simulink model "wind_turbine_modified"  (R2023a)
settings: Solver=VariableStepAuto  StartTime=0.0  StopTime=10.0  RelTol=1e-3
undefined symbols (not defined in the file): F, find_system, Fnom, gcbh, H, ILd_init, ILq_init, Imax_grid_conv, Init, j, Ki_dc_reg, Ki_grid_side_cur_reg, Ki_power_reg, Ki_Q, Ki_rotor_side_cur_reg, Ki_volt_reg, Kp_dc_reg, Kp_grid_side_cur_reg, Kp_power_reg, Kp_Q, Kp_rotor_side_cur_reg, Kp_volt_reg, L_RL, Llr, Lls, p, Pnom, power_A, power_B, power_D, R_RL, Rr, Rs, speed_A, speed_B, speed_C, speed_D, sps_rtmsupport, Vcontrol, Vnom, Wind_On
libraries: simulink_extras x5, spsControlledCurrentSourceLib x4, spsThreePhaseVIMeasurementLib x2, spsWindTurbineDoublyFedInductionGeneratorPhasorTypeLib x1, spsBistableLib x1, spsPower3phPhasorLib x1, spsWindTurbineLib x1
(part 1 of 3)
settings Model: Creator=Adham  LastModifiedBy=Adham

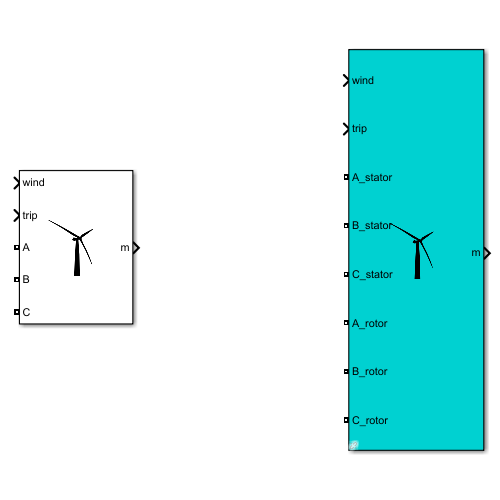
[thumbnail: Simulink's stored preview of the top-level diagram]
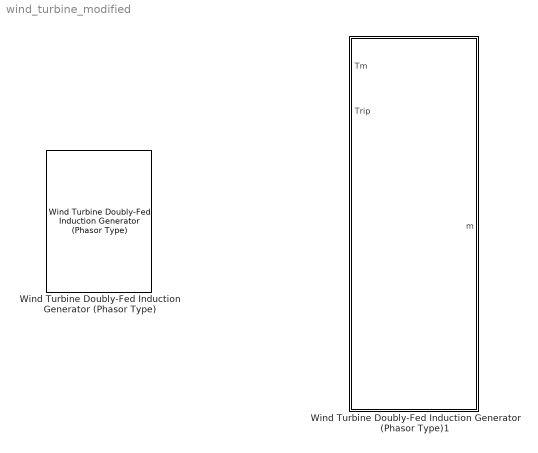
== system wind_turbine_modified ==
  Wind Turbine Doubly-Fed Induction Generator (Phasor Type) : spsWindTurbineDoublyFedInductionGeneratorPhasorTypeLib/Wind Turbine Doubly-Fed Induction Generator (Phasor Type)  ExternalTm=off  nom=[1.5e6/0.9 575 60]  sta=[ 0.00706 0.171]  rot=[ 0.005 0.156]  Lm=2.90  mec=[5.04 0.01 3]  init=[0.2 0 0 0 0 0]  speed_power=[0 0; 0.24 0.007; 0.36 0.024; 0.6 0.112; 0.96 0.46; 1.2 0.898; 1.5 0.898]  Pmec=1.5e6  speed_ABCD=[0.7 0.71 1.2 1.21]  power_C=0.73  wind_point_C=12  pitch_gain=500  pitch_max=45  pitch_rate=2  Pmax=0.5  Lchoke=[0.15 0.15/100]  init_inductor=[0 90]  Vdc_nom=1200  capacitor=10000e-6  ControlVQ=Voltage regulation  Vref=1.0  ExternalVref=off  Qref=0  ExternalQref=on  Iq_ref=0  ExternalIqref=off  Kpi_volt_reg=[1.25 300]  Xs=0.02  Kpi_Q=[0.05 5]  Kpi_power_reg=[1 100]  Kpi_dc_reg=[0.002 0.05]  Kpi_grid_side_cur_reg=[1 100]  Kpi_rotor_side_cur_reg=[0.3 8]  V_slew_rate=100  Q_slew_rate=100  power_slew_rate=1  current_slew_rate=200
      settings: LibrarySourceBlock=|
      | sps_lib/Electrical Machines/Wind Turbine
      | Doubly-Fed Induction Generator
      | (Phasor Type)
  Wind Turbine Doubly-Fed Induction Generator (Phasor Type)1 : Subsystem  AncestorBlock=|  DialogController=POWERSYS.PowerSysDialog  LoadFcn=sps_rtmsupport('LoadFcn',gcbh); %find_system(gcs,'FollowLinks', 'on', 'LookUnderMasks', 'all');  StartFcn=sps_rtmsupport('StartFcn',gcbh);  StopFcn=sps_rtmsupport('StopFcn',gcbh);  mask(Wind Turbine Doubly-Fed Induction Generator (Phasor Type)){ExternalTm=off, nom=[1.5e6/0.9 575 60], sta=[ 0.00706 0.171], rot=[ 0.005 0.156], Lm=2.90, mec=[5.04 0.01 3], init=[0.2 0 0 0 0 0], speed_power=[0 0; 0.24 0.007; 0.36 0.024; 0.6 0.112; 0.96 0.46; 1.2 0.898; 1.5 0.898], Pmec=1.5e6, speed_ABCD=[0.7 0.71 1.2 1.21], power_C=0.73, wind_point_C=12, pitch_gain=500, pitch_max=45, pitch_rate=2, Pmax=0.5, Lchoke=[0.15 0.15/100], init_inductor=[0 90], Vdc_nom=1200, capacitor=10000e-6, ControlVQ=Voltage regulation, Vref=1.0, ExternalVref=off, Qref=0, ExternalQref=on, Iq_ref=0, ExternalIqref=off, Kpi_volt_reg=[1.25 300], Xs=0.02, Kpi_Q=[0.05 5], Kpi_power_reg=[1 100], Kpi_dc_reg=[0.002 0.05], Kpi_grid_side_cur_reg=[1 100], Kpi_rotor_side_cur_reg=[0.3 8], V_slew_rate=100, Q_slew_rate=100, power_slew_rate=1, current_slew_rate=200}
      | sps_lib/Electrical Machines/Wind Turbine
      | Doubly-Fed Induction Generator
      | (Phasor Type)
      mask prompts: ExternalTm "External turbine (Tm mechanical torque input)"; nom "Nominal power, line-to-line voltage, frequency [Pn(VA), Vn(Vrms), fn(Hz)]:"; sta "Stator [Rs, Lls] (pu):"; rot "Rotor [Rr', Llr' ] (pu):"; Lm "Magnetizing inductance Lm (pu):"; mec "Inertia constant, friction factor, and pairs of poles [H(s), F(pu),  p ]:"; init "Initial conditions [s,  th(deg),  Is(pu), ph_Is(deg),  Ir(pu),  ph_Ir(deg)]:"; speed_power "Electric power-speed characteristic: [wr1(pu) p1(pu); wr2(pu) p2(pu); ... ]"; Pmec "Nominal wind turbine mechanical output power (W):"; speed_ABCD "Tracking characteristic speeds: [speed_A(pu) ... speed_D(pu)]"; power_C "Power at point C (pu/mechanical power):"; wind_point_C "Wind speed at point C (m/s):"; pitch_gain "Pitch angle controller gain [Kp]:"; pitch_max "Maximum pitch angle (deg):"; pitch_rate "Maximum rate of change of pitch angle (deg/s):"; Pmax "Converter maximum power (pu):"; Lchoke "Grid-side coupling inductor [L (pu) R (pu)]:"; init_inductor "Coupling inductor initial current: [ IL(pu) ph_IL(deg)]"; Vdc_nom "Nominal DC bus voltage (V):"; capacitor "DC bus capacitor (F):"; ControlVQ "Mode:"; Vref "Reference grid voltage Vref (pu):"; ExternalVref "External"; Qref "Generated reactive power Qref (pu):"; ExternalQref "External"; Iq_ref "Grid-side converter generated reactive current reference (Iq_ref) (pu):"; ExternalIqref "External"; Kpi_volt_reg "Grid voltage regulator gains: [Kp Ki]"; Xs "Droop Xs (pu):"; Kpi_Q "Reactive power regulator gains: [Kp Ki]"; Kpi_power_reg "Power regulator gains: [Kp Ki]"; Kpi_dc_reg "DC bus voltage regulator gains: [Kp Ki]"; Kpi_grid_side_cur_reg "Grid-side converter current regulator gains: [Kp Ki]"; Kpi_rotor_side_cur_reg "Rotor-side converter current regulator gains: [Kp Ki]"; V_slew_rate "Maximum rate of change of reference grid voltage (pu/s):"; Q_slew_rate "Maximum rate of change of reference reactive power (pu/s):"; power_slew_rate "Maximum rate of change of reference power (pu/s):"; current_slew_rate "Maximum rate of change of converter  reference currents (pu/s):"
      mask help: Implements a phasor model of a doubly-fed induction generator driven by a wind turbine.
      mask init:
      | [Pnom,Vnom,Fnom,Rs,Lls,Rr,Llr,H,p,F,Wind_On,FACTSroot,mag_IL_init,ph_IL_init,ILd_init,ILq_init,Imax_grid_conv,speed_A,speed_B,speed_C,speed_D,power_A,power_B,power_D,L_RL,R_RL,Kp_volt_reg,Ki_volt_reg,Kp_Q,Ki_Q,Kp_power_reg,Ki_power_reg,Kp_dc_reg,Ki_dc_reg,Kp_grid_side_cur_reg,Ki_grid_side_cur_reg,Kp_rotor_side_cur_reg,Ki_rotor_side_cur_reg,Vcontrol] ...
      |     = WindTurbineInit (nom,sta,rot,mec,ExternalTm,1,gcbh,Pmax,Lchoke,init_inductor,speed_ABCD,power_C,Kpi_volt_reg,Kpi_Q,Kpi_power_reg,Kpi_dc_reg,Kpi_grid_side_cur_reg,Kpi_rotor_side_cur_reg,ControlVQ);
      settings: CopyFcn=sps_rtmsupport('CopyFcn',gcbh);  DeleteFcn=sps_rtmsupport('DeleteFcn',gcbh);  UndoDeleteFcn=sps_rtmsupport('UndoDeleteFcn',gcbh);  ModelCloseFcn=sps_rtmsupport('ModelCloseFcn',gcbh);  PreSaveFcn=sps_rtmsupport('PreSaveFcn',gcbh);  PostSaveFcn=sps_rtmsupport('PostSaveFcn',gcbh);  NameChangeFcn=sps_rtmsupport('NameChangeFcn',gcbh);  PreCopyFcn=sps_rtmsupport('PreCopyFcn',gcbh);  OpenFcn=sps_rtmsupport('OpenFcn',gcbh, [1 21,23,25,27]);  CloseFcn=sps_rtmsupport('CloseFcn',gcbh);  PreDeleteFcn=sps_rtmsupport('PreDeleteFcn',gcbh);
      settings: LibrarySourceBlock=|
      | sps_lib/Electrical Machines/Wind Turbine
      | Doubly-Fed Induction Generator
      | (Phasor Type)
      mask Help: helpview(psbhelp)
      mask Callback ExternalTm: WindTurbineCback(gcbh);
      mask TypeOptions ControlVQ: Voltage regulation | Var regulation
      mask Callback ControlVQ: WindTurbineCback(gcbh);
      mask Callback ExternalVref: WindTurbineCback(gcbh);
      mask Callback ExternalQref: WindTurbineCback(gcbh);
      mask Callback ExternalIqref: WindTurbineCback(gcbh);
      mask DialogControl generatordata Prompt: Generator
      mask DialogControl turbinedata Prompt: Turbine
      mask DialogControl Display Prompt: Display wind turbine power characteristics
      mask DialogControl Display Callback: WindTurbineDisplay(gcbh);
      mask DialogControl convertersdata Prompt: Converters
      mask DialogControl controlparameters Prompt: Control
      mask Display:
      | port_label('LConn',1,'A_stator')
      | port_label('LConn',2,'B_stator')
      | port_label('LConn',3,'C_stator')
      | port_label('LConn',4,'A_rotor')
      | port_label('LConn',5,'B_rotor')
      | port_label('LConn',6,'C_rotor')
      | 
      | port_label('output',1,'m')
      | 
      | Block = gcbh;
      | switch get_param(Block,'ExternalTm')
      |     case 'on'
      |         port_label('input',1,'Tm')
      |     case 'off'
      |         port_label('input',1,'wind')
      | end
      | 
      | x = 2;
      | 
      | switch get_param(Block,'ControlVQ')
      |     case 'Voltage regulation'
      |         switch get_param(Block,'ExternalVref')
      |             case 'on'
      |                 port_label('input',2,'Vref');
      |                 x = 3;
      |         end
      |     case 'Var regulation'
      |         switch get_param(Block,'ExternalQref')
      |             case 'on'
      |                 port_label('input',2,'Qref');
      |                 x = 3;
      |         end
      | end
      | 
      | switch get_param(Block,'ExternalIqref')
      |     case 'on'
      |         port_label('input',x,'Iq_ref');
      |         x = x +1;
      | end
      | 
      | port_label('input',x,'trip');

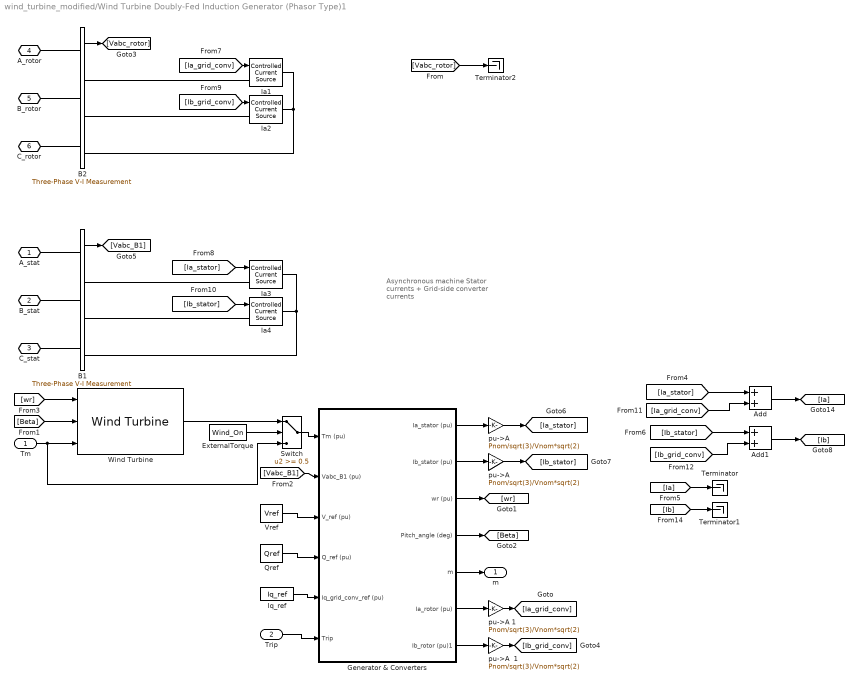
== system wind_turbine_modified/Wind Turbine Doubly-Fed Induction Generator (Phasor Type)1 ==
  note: Asynchronous machine
      | Stator currents
      | +
      | Grid-side converter
      | currents
  "Tm " : Inport
  Trip : Inport  Port=2
  Add : Sum
  Add1 : Sum
  B1 : spsThreePhaseVIMeasurementLib/Three-Phase V-I Measurement  VoltageMeasurement=phase-to-ground  SetLabelV=off  LabelV=Vabc_B1  Vpu=on  VpuLL=off  CurrentMeasurement=no  SetLabelI=off  LabelI=Iabc_Beol  Ipu=off  Pbase=Pnom  Vbase=Vnom  OutputType=Complex  PhasorSimulation=on  PSBequivalent=0
  B2 : spsThreePhaseVIMeasurementLib/Three-Phase V-I Measurement  VoltageMeasurement=phase-to-ground  SetLabelV=off  LabelV=Vabc_B1  Vpu=on  VpuLL=off  CurrentMeasurement=no  SetLabelI=off  LabelI=Iabc_Beol  Ipu=off  Pbase=Pnom  Vbase=Vnom  OutputType=Complex  PhasorSimulation=on  PSBequivalent=0
  ExternalTorque : Constant  Value=Wind_On
  Generator & Converters : Subsystem
  Ia{1..4} (4 alike) : spsControlledCurrentSourceLib/Controlled Current Source  Description=source block  Initialize=off  Source_Type=AC  Amplitude=0  Phase=0  Frequency=0  Measurements=None
  "Iq_ref " : Constant  Value=Iq_ref
  "Qref " : Constant  Value=Qref
  Switch : Switch  Threshold=0.5  InputSameDT=off
  Terminator : Terminator
  Terminator1 : Terminator
  Terminator2 : Terminator
  "Vref " : Constant  Value=Vref
  Wind Turbine : spsWindTurbineLib/Wind Turbine  Pnom=Pmec  Pelec_base=Pnom  wind_base=wind_point_C  P_wind_base=power_C  speed_nom=speed_C  pitch_angle=0  c1_c6="[0.51763          116          0.4            5           21     0.006795]"  cp_nom=0.48  lambda_nom=8.1
  "pu->A " : Gain  Gain=Pnom/sqrt(3)/Vnom*sqrt(2)  SaturateOnIntegerOverflow=on  OutDataTypeStr=Inherit: Same as input  ParamDataTypeStr=Inherit: Same as input
  "pu->A  " : Gain  Gain=Pnom/sqrt(3)/Vnom*sqrt(2)  SaturateOnIntegerOverflow=on  OutDataTypeStr=Inherit: Same as input  ParamDataTypeStr=Inherit: Same as input
  pu->A  1 : Gain  Gain=Pnom/sqrt(3)/Vnom*sqrt(2)  SaturateOnIntegerOverflow=on  OutDataTypeStr=Inherit: Same as input  ParamDataTypeStr=Inherit: Same as input
  pu->A 1 : Gain  Gain=Pnom/sqrt(3)/Vnom*sqrt(2)  SaturateOnIntegerOverflow=on  OutDataTypeStr=Inherit: Same as input  ParamDataTypeStr=Inherit: Same as input
  A_stat : PMIOPort  Side=Left
  B_stat : PMIOPort  Port=2  Side=Left
  C_stat : PMIOPort  Port=3  Side=Left
  A_rotor : PMIOPort  Port=4  Side=Left
  B_rotor : PMIOPort  Port=5  Side=Left
  C_rotor : PMIOPort  Port=6  Side=Left
  m : Outport  VectorParamsAs1DForOutWhenUnconnected=off
  wires:
  Switch/1 -> Generator & Converters/1(Tm (pu))
  [Vabc_B1] -> Generator & Converters/2(Vabc_B1 (pu))
  Generator & Converters/1(Ia_stator (pu)) -> "pu->A "/1
  "pu->A  "/1 -> [Ib_stator]
  "pu->A "/1 -> [Ia_stator]
  B1/1 -> [Vabc_B1]
  Generator & Converters/3(wr (pu)) -> [wr]
  ExternalTorque/1 -> Switch/2
  Generator & Converters/2(Ib_stator (pu)) -> "pu->A  "/1
  "Tm "/1 -> Wind Turbine/3, Switch/3
  [wr] -> Wind Turbine/1
  Wind Turbine/1 -> Switch/1
  Generator & Converters/5(m) -> m/1
  "Qref "/1 -> Generator & Converters/4(Q_ref (pu))
  "Iq_ref "/1 -> Generator & Converters/5(Iq_grid_conv_ref (pu))
  "Vref "/1 -> Generator & Converters/3(V_ref (pu))
  [Ia_stator] -> Ia3/1
  [Ib_stator] -> Ia4/1
  Trip/1 -> Generator & Converters/6(Trip)
  [Beta] -> Wind Turbine/2
  Generator & Converters/4(Pitch_angle (deg)) -> [Beta]
  B2/1 -> [Vabc_rotor]
  [Ia_grid_conv] -> Ia1/1
  [Ib_grid_conv] -> Ia2/1
  Generator & Converters/7(Ib_rotor (pu)1) -> pu->A  1/1
  Generator & Converters/6(Ia_rotor (pu)) -> pu->A 1/1
  Add1/1 -> [Ib]
  Add/1 -> [Ia]
  pu->A 1/1 -> [Ia_grid_conv]
  pu->A  1/1 -> [Ib_grid_conv]
  [Ib_grid_conv] -> Add1/2
  [Ib_stator] -> Add1/1
  [Ia_grid_conv] -> Add/2
  [Ia_stator] -> Add/1
  [Ia] -> Terminator/1
  [Ib] -> Terminator1/1
  [Vabc_rotor] -> Terminator2/1
  connections:
  B_stat/RConn1 -- B1/LConn2
  C_stat/RConn1 -- B1/LConn3
  Ia4/LConn1 -- B1/RConn2
  A_stat/RConn1 -- B1/LConn1
  Ia3/LConn1 -- B1/RConn1
  B2/RConn2 -- Ia2/LConn1
  Ia1/LConn1 -- B2/RConn1
  B2/LConn3 -- C_rotor/RConn1
  B1/RConn3 -- Ia3/RConn1 -- Ia4/RConn1
  B2/LConn2 -- B_rotor/RConn1
  A_rotor/RConn1 -- B2/LConn1
  Ia1/RConn1 -- B2/RConn3 -- Ia2/RConn1

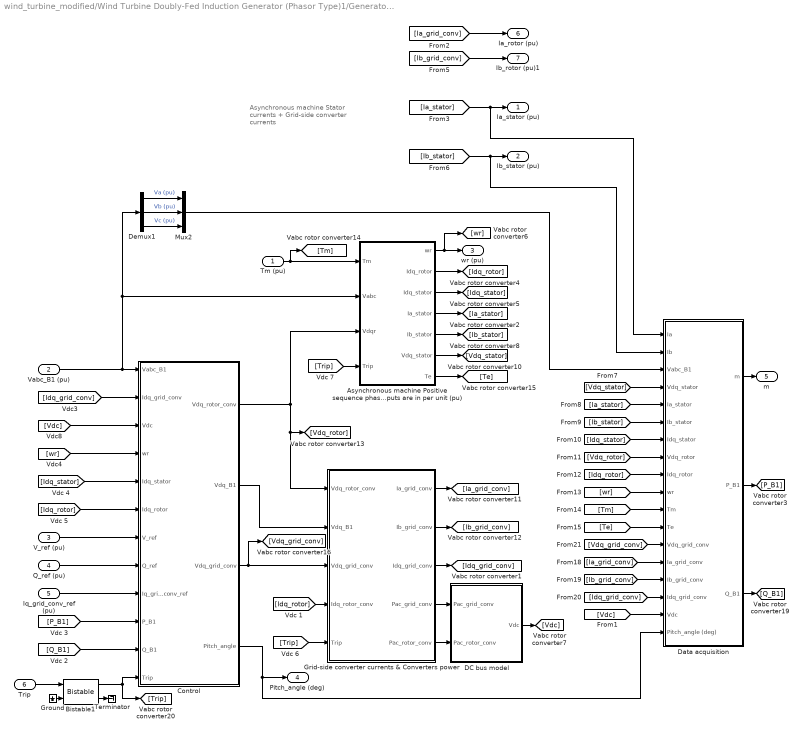
== system wind_turbine_modified/Wind Turbine Doubly-Fed Induction Generator (Phasor Type)1/Generator & Converters ==
  note: Asynchronous machine
      | Stator currents
      | +
      | Grid-side converter
      | currents
  Tm (pu) : Inport
  Vabc_B1 (pu) : Inport  Port=2
  V_ref (pu) : Inport  Port=3
  Q_ref (pu) : Inport  Port=4
  Iq_grid_conv_ref (pu) : Inport  Port=5
  Trip : Inport  Port=6
  Asynchronous machine Positive sequence phasor model Inputs and outputs are in per unit (pu) : Subsystem  mask(Asynchronous Machine Model){nom=[ Pnom Vnom Fnom ], sta=[ Rs Lls], rot=[ Rr Llr], Lm=Lm, mec=[H F p], ini=init}
      mask prompts: nom "Nom. power,L-L volt. and freq. [ Pn(VA),Vn(Vrms),fn(Hz) ]:"; sta "Stator [ Rs,Lls (pu) ]:"; rot "Rotor [ Rr',Llr' (pu) ]:"; Lm "Magnetizing inductance Lm (pu):"; mec "Inertia constant,friction factor and pairs of poles [ H(s)  F(pu)  p() ]:"; ini "Initial conditions [s()  th(deg)  Is(pu)  ph_Is(deg)  Ir(pu)  ph_Ir(deg)]:"
      mask help: Implements a three-phase asynchronous machine (wound rotor) modelled in the dq stator reference frame. Stator and rotor windings are connected in wye to an internal neutral point.
      mask init:
      | %Initializes the Asynchronous Machine block before simulation.
      | 
      | % Base angular frequency
      | web=nom(3)*2*pi;
      | 
      | Rs=sta(1); Lls=sta(2);		% stator resistance and leakage inductance
      | Rr=rot(1); Llr=rot(2);		% rotor resistance and leakage inductance
      | Lm=Lm(1);			        % mutual inductance
      | H=mec(1); F=mec(2); p=mec(3);	% inertia, friction and pole pairs
      | s=ini(1);			% initial slip
      | wmo=1-s;			% initial speed
      | tho=ini(2)*pi/180;		% initial rotor angle
      | 
      | iso_mag=ini(3); iso_ph=ini(4)*pi/180; % init. stator current, phase A
      | iro_mag=ini(5); iro_ph=ini(6)*pi/180; % init. rotor current, phase A
      | 
      | % conversion of initial stator and rotor currents from polar to rectangular
      | % coordinates
      | [isdo,isqo]=pol2cart(iso_ph,iso_mag);
      | [irdo,irqo]=pol2cart(iro_ph,iro_mag);
      | 
      | % Initial fluxes (pu): inductances in pu, currents in pu
      | phisqo=((Lls+Lm)*isqo+Lm*irqo);
      | phisdo=((Lls+Lm)*isdo+Lm*irdo);
      | phirqo=((Llr+Lm)*irqo+Lm*isqo);
      | phirdo=((Llr+Lm)*irdo+Lm*isdo);
      | 
      | % Other inductances -------------------------------------------------------
      | 
      | Laq=1/(1/Lm+1/Lls+1/Llr);
      | Lad=Laq;
      mask Help: First 3 inputs: Stator terminals = phases a, b and c; 4th input: Simulink signal = Mechanical torque applied to the shaft (pu, >0 for motor mode, <0 for generator mode); First 3 outputs: Rotor terminals = phases a, b and c; 4th output: Simulink measurement output = vector (20x1) containing the following (all currents flowing into the machine): [1-3] : Rotor line currents ira, irb and irc; [4-5] : Rotor currents iqr and idr; [6-7] : Rotor fluxes phiqr and  phidr; [8-9] : Rotor voltages vqr and vdr; [10-12] : Stator line currents isa, isb, isc; [13-14] : Stator currents iqs and ids; [15-16] : Stator fluxes phiqs and  phids; [17-18] : Stator voltages vqs and vds; [19] : Rotor speed wm; [20 ]: Electromagnetic torque Te. Units of output measurement depend on checkbox in block's dialog box.
  Bistable1 : spsBistableLib/Bistable  Qpriority=Set  ic=0  Ts=0
      settings: LibrarySourceBlock=sps_lib/Control/Bistable
  Control : Subsystem
  DC bus model : Subsystem  mask(DC bus model){Pnom=Pnom, C=capacitor, Vdc_Init=Vdc_nom}
      mask prompts: Pnom "Nominal power (W):"; C "Capacitor (F):"; Vdc_Init "Initial voltage (V):"
  Data acquisition : Subsystem
  Demux1 : Demux  Outputs=3
      settings: DisplayOption=none
  Grid-side converter currents & Converters power : Subsystem
  Ground : Ground
  Mux2 : Mux  Inputs=3
  Terminator : Terminator
  Ia_stator (pu) : Outport  VectorParamsAs1DForOutWhenUnconnected=off
  Ib_stator (pu) : Outport  Port=2  VectorParamsAs1DForOutWhenUnconnected=off
  wr (pu) : Outport  Port=3  VectorParamsAs1DForOutWhenUnconnected=off
  Pitch_angle (deg) : Outport  Port=4  VectorParamsAs1DForOutWhenUnconnected=off
  m : Outport  Port=5  VectorParamsAs1DForOutWhenUnconnected=off
  Ia_rotor (pu) : Outport  Port=6  VectorParamsAs1DForOutWhenUnconnected=off
  Ib_rotor (pu)1 : Outport  Port=7  VectorParamsAs1DForOutWhenUnconnected=off
  wires:
  DC bus model/1(Vdc) -> [Vdc]
  [Idq_rotor] -> Control/6(Idq_rotor)
  [Idq_stator] -> Control/5(Idq_stator)
  [Vdc] -> Control/3(Vdc)
  [wr] -> Control/4(wr)
  Control/3(Vdq_grid_conv) -> Grid-side converter currents & Converters power/3(Vdq_grid_conv), [Vdq_grid_conv]
  Control/1(Vdq_rotor_conv) -> Asynchronous machine Positive sequence phasor model Inputs and outputs are in per unit (pu)/3("Vdqr "), Grid-side converter currents & Converters power/1(Vdq_rotor_conv), [Vdq_rotor]
  Control/2(Vdq_B1) -> Grid-side converter currents & Converters power/2(Vdq_B1)
  Grid-side converter currents & Converters power/3(Idq_grid_conv) -> [Idq_grid_conv]
  [Idq_grid_conv] -> Control/2(Idq_grid_conv)
  Asynchronous machine Positive sequence phasor model Inputs and outputs are in per unit (pu)/3(Idq_stator) -> [Idq_stator]
  Asynchronous machine Positive sequence phasor model Inputs and outputs are in per unit (pu)/2(Idq_rotor) -> [Idq_rotor]
  Tm (pu)/1 -> Asynchronous machine Positive sequence phasor model Inputs and outputs are in per unit (pu)/1(Tm), [Tm]
  Asynchronous machine Positive sequence phasor model Inputs and outputs are in per unit (pu)/5(Ib_stator) -> [Ib_stator]
  Asynchronous machine Positive sequence phasor model Inputs and outputs are in per unit (pu)/4(Ia_stator) -> [Ia_stator]
  [Idq_rotor] -> Grid-side converter currents & Converters power/4(Idq_rotor_conv)
  Grid-side converter currents & Converters power/4(Pac_grid_conv) -> DC bus model/1(Pac_grid_conv)
  Grid-side converter currents & Converters power/5(Pac_rotor_conv) -> DC bus model/2(Pac_rotor_conv)
  Vabc_B1 (pu)/1 -> Control/1(Vabc_B1), Asynchronous machine Positive sequence phasor model Inputs and outputs are in per unit (pu)/2(Vabc), Demux1/1
  [Ia_stator] -> Ia_stator (pu)/1, Data acquisition/1(Ia)
  [Ib_stator] -> Ib_stator (pu)/1, Data acquisition/2(Ib)
  Asynchronous machine Positive sequence phasor model Inputs and outputs are in per unit (pu)/1(wr) -> wr (pu)/1, [wr]
  Asynchronous machine Positive sequence phasor model Inputs and outputs are in per unit (pu)/6(Vdq_stator) -> [Vdq_stator]
  Grid-side converter currents & Converters power/1(Ia_grid_conv) -> [Ia_grid_conv]
  Grid-side converter currents & Converters power/2(Ib_grid_conv) -> [Ib_grid_conv]
  [Ia_grid_conv] -> Ia_rotor (pu)/1
  [Ib_grid_conv] -> Ib_rotor (pu)1/1
  Asynchronous machine Positive sequence phasor model Inputs and outputs are in per unit (pu)/7(Te) -> [Te]
  [Idq_grid_conv] -> Data acquisition/16(Idq_grid_conv)
  [Ib_grid_conv] -> Data acquisition/15(Ib_grid_conv)
  [Ia_grid_conv] -> Data acquisition/14(Ia_grid_conv)
  [Vdq_grid_conv] -> Data acquisition/13(Vdq_grid_conv)
  [Te] -> Data acquisition/12(Te)
  [Tm] -> Data acquisition/11(Tm)
  [wr] -> Data acquisition/10(wr)
  [Idq_rotor] -> Data acquisition/9(Idq_rotor)
  [Vdq_rotor] -> Data acquisition/8(Vdq_rotor)
  [Idq_stator] -> Data acquisition/7(Idq_stator)
  [Ib_stator] -> Data acquisition/6(Ib_stator)
  [Ia_stator] -> Data acquisition/5(Ia_stator)
  [Vdq_stator] -> Data acquisition/4(Vdq_stator)
  Data acquisition/1(m) -> m/1
  [Vdc] -> Data acquisition/17(Vdc)
  Demux1/1 -> Mux2/1  "Va (pu)"
  Demux1/2 -> Mux2/2  "Vb (pu)"
  Mux2/1 -> Data acquisition/3(Vabc_B1)
  Demux1/3 -> Mux2/3  "Vc (pu)"
  Data acquisition/3(Q_B1) -> [Q_B1]
  Q_ref (pu)/1 -> Control/8(Q_ref)
  Iq_grid_conv_ref (pu)/1 -> Control/9(Iq_grid_conv_ref)
  Data acquisition/2(P_B1) -> [P_B1]
  [P_B1] -> Control/10(P_B1)
  [Q_B1] -> Control/11(Q_B1)
  V_ref (pu)/1 -> Control/7(V_ref)
  [Trip] -> Grid-side converter currents & Converters power/5(Trip)
  [Trip] -> Asynchronous machine Positive sequence phasor model Inputs and outputs are in per unit (pu)/4(Trip)
  Trip/1 -> Bistable1/1
  Bistable1/2 -> Terminator/1
  Ground/1 -> Bistable1/2
  Bistable1/1 -> [Trip], Control/12(Trip)
  Control/4(Pitch_angle) -> Data acquisition/18(Pitch_angle (deg)), Pitch_angle (deg)/1

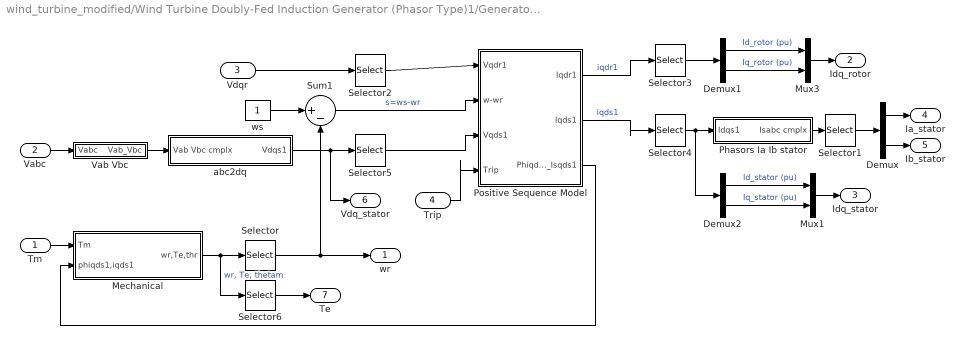
== system wind_turbine_modified/Wind Turbine Doubly-Fed Induction Generator (Phasor Type)1/Generator & Converters/Asynchronous machine Positive sequence phasor model Inputs and outputs are in per unit (pu) ==
  Tm : Inport
  Vabc : Inport  Port=2
  "Vdqr " : Inport  Port=3
  Trip : Inport  Port=4
  Demux : Demux  Outputs=2
      settings: DisplayOption=none
  Demux1 : Demux  Outputs=2
      settings: DisplayOption=none
  Demux2 : Demux  Outputs=2
      settings: DisplayOption=none
  Mechanical : Subsystem
  Mux1 : Mux  Inputs=2
  Mux3 : Mux  Inputs=2
  Phasors Ia Ib stator : Subsystem
  Positive Sequence Model : Subsystem
  Selector : Selector  InputPortWidth=3  IndexOptions=Index vector (dialog)  Indices=1  OutputSizes=1
  Selector1 : Selector  InputPortWidth=3  IndexOptions=Index vector (dialog)  Indices=[1 2]  OutputSizes=1
  Selector{2..5} (4 alike) : Selector  InputPortWidth=2  IndexOptions=Index vector (dialog)  Indices=[2 1]  OutputSizes=1
  Selector6 : Selector  InputPortWidth=3  IndexOptions=Index vector (dialog)  Indices=2  OutputSizes=1
  Sum1 : Sum  Inputs=|+-  InputSameDT=on  SaturateOnIntegerOverflow=on  OutDataTypeStr=Inherit: Same as first input
  Vab Vbc : Subsystem
  abc2dq : Subsystem
  ws : Constant
  wr : Outport  VectorParamsAs1DForOutWhenUnconnected=off
  Idq_rotor : Outport  Port=2  VectorParamsAs1DForOutWhenUnconnected=off
  Idq_stator : Outport  Port=3  VectorParamsAs1DForOutWhenUnconnected=off
  Ia_stator : Outport  Port=4  VectorParamsAs1DForOutWhenUnconnected=off
  Ib_stator : Outport  Port=5  VectorParamsAs1DForOutWhenUnconnected=off
  Vdq_stator : Outport  Port=6  VectorParamsAs1DForOutWhenUnconnected=off
  Te : Outport  Port=7  VectorParamsAs1DForOutWhenUnconnected=off
  wires:
  Selector4/1 -> Phasors Ia Ib stator/1(Idqs1), Demux2/1
  Selector5/1 -> Positive Sequence Model/3(Vqds1)
  Selector2/1 -> Positive Sequence Model/1(Vqdr1)
  Sum1/1 -> Positive Sequence Model/2(w-wr)  "s=ws-wr"
  Selector/1 -> wr/1, Sum1/2
  ws/1 -> Sum1/1
  Mechanical/1(wr,Te,thr) -> Selector/1, Selector6/1  "wr, Te, thetam"
  "Vdqr "/1 -> Selector2/1
  abc2dq/1(Vdqs1) -> Selector5/1, Vdq_stator/1
  Vab Vbc/1(Vab_Vbc) -> abc2dq/1(Vab Vbc cmplx)
  Vabc/1 -> Vab Vbc/1(Vabc)
  Phasors Ia Ib stator/1(Isabc cmplx) -> Selector1/1
  Tm/1 -> Mechanical/1(Tm)
  Demux/1 -> Ia_stator/1
  Demux/2 -> Ib_stator/1
  Selector1/1 -> Demux/1
  Selector6/1 -> Te/1
  Selector3/1 -> Demux1/1
  Demux1/1 -> Mux3/1  "Id_rotor (pu)"
  Demux1/2 -> Mux3/2  "Iq_rotor (pu)"
  Mux3/1 -> Idq_rotor/1
  Demux2/1 -> Mux1/1  "Id_stator (pu)"
  Demux2/2 -> Mux1/2  "Iq_stator (pu)"
  Mux1/1 -> Idq_stator/1
  Positive Sequence Model/1(Iqdr1) -> Selector3/1  "iqdr1"
  Positive Sequence Model/2(Iqds1) -> Selector4/1  "iqds1"
  Positive Sequence Model/3(Phiqds1_Isqds1) -> Mechanical/2(phiqds1,iqds1)
  Trip/1 -> Positive Sequence Model/4(Trip)

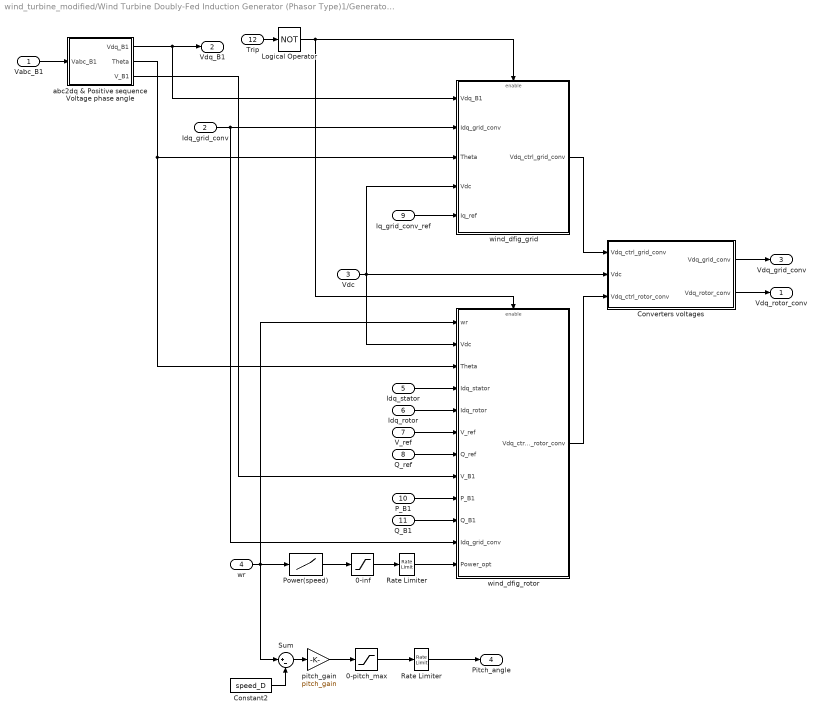
== system wind_turbine_modified/Wind Turbine Doubly-Fed Induction Generator (Phasor Type)1/Generator & Converters/Control ==
  Vabc_B1 : Inport
  Idq_grid_conv : Inport  Port=2
  Vdc : Inport  Port=3
  wr : Inport  Port=4
  Idq_stator : Inport  Port=5
  Idq_rotor : Inport  Port=6
  V_ref : Inport  Port=7  SampleTime=0
  Q_ref : Inport  Port=8  SampleTime=0
  Iq_grid_conv_ref : Inport  Port=9  SampleTime=0
  P_B1 : Inport  Port=10
  Q_B1 : Inport  Port=11
  Trip : Inport  Port=12
  0-inf : Saturate  UpperLimit=inf  LowerLimit=0
  0-pitch_max : Saturate  UpperLimit=pitch_max  LowerLimit=0
  Constant2 : Constant  Value=speed_D
  Converters voltages : Subsystem
  Logical Operator : Logic  Operator=NOT  AllPortsSameDT=off  OutDataTypeStr=float('double')  SampleTime=0
  Power(speed) : Lookup_n-D  NumberOfTableDimensions=1  BreakpointsForDimension1=speed_power(:,1)  Table=speed_power(:,2)  InternalRulePriority=Speed  RndMeth=Simplest
  "Rate Limiter " : RateLimiter  RisingSlewLimit=power_slew_rate  FallingSlewLimit=-power_slew_rate
  "Rate Limiter   " : RateLimiter  RisingSlewLimit=pitch_rate  FallingSlewLimit=-pitch_rate
  Sum : Sum  Inputs=|+-  SaturateOnIntegerOverflow=on
  abc2dq & Positive sequence Voltage phase angle : Subsystem
  pitch_gain : Gain  Gain=pitch_gain  SaturateOnIntegerOverflow=on  OutDataTypeStr=Inherit: Same as input  ParamDataTypeStr=Inherit: Same as input
  wind_dfig_grid : Subsystem
  wind_dfig_rotor : Subsystem
  Vdq_rotor_conv : Outport  VectorParamsAs1DForOutWhenUnconnected=off
  Vdq_B1 : Outport  Port=2  VectorParamsAs1DForOutWhenUnconnected=off
  Vdq_grid_conv : Outport  Port=3  VectorParamsAs1DForOutWhenUnconnected=off
  Pitch_angle : Outport  Port=4  VectorParamsAs1DForOutWhenUnconnected=off
  wires:
  Vdc/1 -> Converters voltages/2(Vdc), wind_dfig_grid/4(Vdc), wind_dfig_rotor/2(Vdc)
  abc2dq & Positive sequence Voltage phase angle/2(Theta) -> wind_dfig_grid/3(Theta), wind_dfig_rotor/3(Theta)
  abc2dq & Positive sequence Voltage phase angle/1(Vdq_B1) -> Vdq_B1/1, wind_dfig_grid/1(Vdq_B1)
  Converters voltages/2(Vdq_rotor_conv) -> Vdq_rotor_conv/1
  Converters voltages/1(Vdq_grid_conv) -> Vdq_grid_conv/1
  Idq_grid_conv/1 -> wind_dfig_grid/2(Idq_grid_conv), wind_dfig_rotor/11(Idq_grid_conv)
  Vabc_B1/1 -> abc2dq & Positive sequence Voltage phase angle/1(Vabc_B1)
  Iq_grid_conv_ref/1 -> wind_dfig_grid/5(Iq_ref)
  Idq_stator/1 -> wind_dfig_rotor/4(Idq_stator)
  Idq_rotor/1 -> wind_dfig_rotor/5(Idq_rotor)
  V_ref/1 -> wind_dfig_rotor/6(V_ref)
  Q_ref/1 -> wind_dfig_rotor/7(Q_ref)
  abc2dq & Positive sequence Voltage phase angle/3(V_B1) -> wind_dfig_rotor/8(V_B1)
  wr/1 -> Power(speed)/1, Sum/1, wind_dfig_rotor/1(wr)
  P_B1/1 -> wind_dfig_rotor/9(P_B1)
  Q_B1/1 -> wind_dfig_rotor/10(Q_B1)
  Trip/1 -> Logical Operator/1
  wind_dfig_grid/1(Vdq_ctrl_grid_conv) -> Converters voltages/1(Vdq_ctrl_grid_conv)
  0-inf/1 -> "Rate Limiter "/1
  Power(speed)/1 -> 0-inf/1
  "Rate Limiter "/1 -> wind_dfig_rotor/12(Power_opt)
  0-pitch_max/1 -> "Rate Limiter   "/1
  Constant2/1 -> Sum/2
  Sum/1 -> pitch_gain/1
  pitch_gain/1 -> 0-pitch_max/1
  "Rate Limiter   "/1 -> Pitch_angle/1
  wind_dfig_rotor/1(Vdq_ctrl_rotor_conv) -> Converters voltages/3(Vdq_ctrl_rotor_conv)
  Logical Operator/1 -> wind_dfig_grid/Enable, wind_dfig_rotor/Enable

== system wind_turbine_modified/Wind Turbine Doubly-Fed Induction Generator (Phasor Type)1/Generator & Converters/DC bus model ==
  note: Pdc = Pac_grid_conv - Pac_rotor_conv
  Pac_grid_conv : Inport
  Pac_rotor_conv : Inport  Port=2
  Integrator : Integrator  InitialCondition=Vdc_Init  LowerSaturationLimit=1e-6  ZeroCross=off
  Product2 : Product  Inputs=*/  InputSameDT=on  SaturateOnIntegerOverflow=on  OutDataTypeStr=Inherit: Same as first input
  Sum2 : Sum  Inputs=|+-  InputSameDT=on  SaturateOnIntegerOverflow=on  OutDataTypeStr=Inherit: Same as first input
  deg->rad1 : Gain  Gain=1/C  SaturateOnIntegerOverflow=on  OutDataTypeStr=Inherit: Same as input  ParamDataTypeStr=Inherit: Same as input
  pu->W : Gain  Gain=Pnom  SaturateOnIntegerOverflow=on  OutDataTypeStr=Inherit: Same as input  ParamDataTypeStr=Inherit: Same as input
  Vdc : Outport  VectorParamsAs1DForOutWhenUnconnected=off
  wires:
  pu->W/1 -> Product2/1
  Pac_grid_conv/1 -> Sum2/1
  deg->rad1/1 -> Integrator/1
  Integrator/1 -> Vdc/1, Product2/2  "Vdc"
  Product2/1 -> deg->rad1/1  "Idc"
  Pac_rotor_conv/1 -> Sum2/2
  Sum2/1 -> pu->W/1

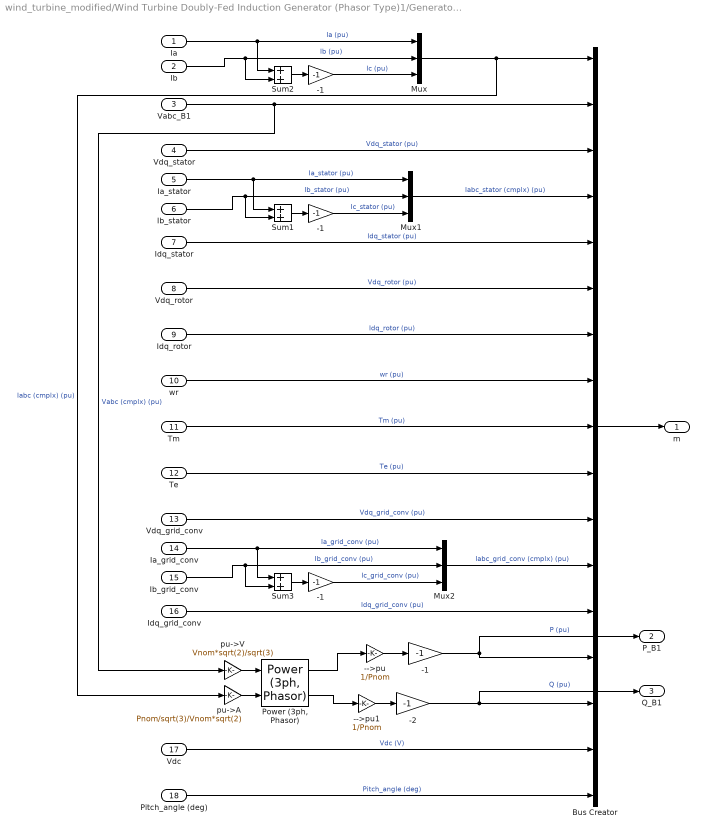
== system wind_turbine_modified/Wind Turbine Doubly-Fed Induction Generator (Phasor Type)1/Generator & Converters/Data acquisition ==
  Ia : Inport
  Ib : Inport  Port=2
  Vabc_B1 : Inport  Port=3
  Vdq_stator : Inport  Port=4
  Ia_stator : Inport  Port=5
  Ib_stator : Inport  Port=6
  Idq_stator : Inport  Port=7
  Vdq_rotor : Inport  Port=8
  Idq_rotor : Inport  Port=9
  wr : Inport  Port=10
  Tm : Inport  Port=11
  Te : Inport  Port=12
  Vdq_grid_conv : Inport  Port=13
  Ia_grid_conv : Inport  Port=14
  Ib_grid_conv : Inport  Port=15
  Idq_grid_conv : Inport  Port=16
  Vdc : Inport  Port=17
  Pitch_angle (deg) : Inport  Port=18
  " -1" : Gain  Gain=-1  SaturateOnIntegerOverflow=on  OutDataTypeStr=Inherit: Same as input  ParamDataTypeStr=Inherit: Same as input
  -->pu : Gain  Gain=1/Pnom  SaturateOnIntegerOverflow=on  OutDataTypeStr=Inherit: Same as input  ParamDataTypeStr=Inherit: Same as input
  -->pu1 : Gain  Gain=1/Pnom  SaturateOnIntegerOverflow=on  OutDataTypeStr=Inherit: Same as input  ParamDataTypeStr=Inherit: Same as input
  -1 : Gain  Gain=-1  SaturateOnIntegerOverflow=on  OutDataTypeStr=Inherit: Same as input  ParamDataTypeStr=Inherit: Same as input
  "-1 " : Gain  Gain=-1  SaturateOnIntegerOverflow=on  OutDataTypeStr=Inherit: Same as input  ParamDataTypeStr=Inherit: Same as input
  "-1  " : Gain  Gain=-1  SaturateOnIntegerOverflow=on  OutDataTypeStr=Inherit: Same as input  ParamDataTypeStr=Inherit: Same as input
  -2 : Gain  Gain=-1  SaturateOnIntegerOverflow=on  OutDataTypeStr=Inherit: Same as input  ParamDataTypeStr=Inherit: Same as input
  Bus Creator : BusCreator  Inputs=17
  Mux : Mux  Inputs=3
  Mux1 : Mux  Inputs=3
  Mux2 : Mux  Inputs=3
  "Power (3ph, Phasor)" : spsPower3phPhasorLib/Power (3ph, Phasor)
      settings: LibrarySourceBlock=|
      | sps_lib/Sensors and Measurements/Power
      | (3ph, Phasor)
  Sum1 : Sum  SaturateOnIntegerOverflow=on
  Sum2 : Sum  SaturateOnIntegerOverflow=on
  Sum3 : Sum  SaturateOnIntegerOverflow=on
  pu->A : Gain  Gain=Pnom/sqrt(3)/Vnom*sqrt(2)  SaturateOnIntegerOverflow=on  OutDataTypeStr=Inherit: Same as input  ParamDataTypeStr=Inherit: Same as input
  pu->V : Gain  Gain=Vnom*sqrt(2)/sqrt(3)  SaturateOnIntegerOverflow=on  OutDataTypeStr=Inherit: Same as input  ParamDataTypeStr=Inherit: Same as input
  m : Outport  VectorParamsAs1DForOutWhenUnconnected=off
  P_B1 : Outport  Port=2  VectorParamsAs1DForOutWhenUnconnected=off
  Q_B1 : Outport  Port=3  VectorParamsAs1DForOutWhenUnconnected=off
  wires:
  pu->A/1 -> "Power (3ph, Phasor)"/2
  -->pu/1 -> -1/1
  Sum2/1 -> "-1 "/1
  "-1 "/1 -> Mux/3  "Ic (pu)"
  Ib/1 -> Sum2/2, Mux/2  "Ib (pu)"
  Ia/1 -> Sum2/1, Mux/1  "Ia (pu)"
  Sum1/1 -> "-1  "/1
  "-1  "/1 -> Mux1/3  "Ic_stator (pu)"
  Ib_stator/1 -> Mux1/2, Sum1/2  "Ib_stator (pu)"
  Ia_stator/1 -> Mux1/1, Sum1/1  "Ia_stator (pu)"
  pu->V/1 -> "Power (3ph, Phasor)"/1
  Sum3/1 -> " -1"/1
  " -1"/1 -> Mux2/3  "Ic_grid_conv (pu)"
  Ib_grid_conv/1 -> Sum3/2, Mux2/2  "Ib_grid_conv (pu)"
  Ia_grid_conv/1 -> Sum3/1, Mux2/1  "Ia_grid_conv (pu)"
  Mux1/1 -> Bus Creator/4  "Iabc_stator (cmplx) (pu)"
  Mux/1 -> pu->A/1, Bus Creator/1  "Iabc (cmplx) (pu)"
  Vabc_B1/1 -> pu->V/1, Bus Creator/2  "Vabc (cmplx) (pu)"
  Vdq_stator/1 -> Bus Creator/3  "Vdq_stator (pu)"
  Idq_stator/1 -> Bus Creator/5  "Idq_stator (pu)"
  Vdq_rotor/1 -> Bus Creator/6  "Vdq_rotor (pu)"
  Idq_rotor/1 -> Bus Creator/7  "Idq_rotor (pu)"
  wr/1 -> Bus Creator/8  "wr (pu)"
  Tm/1 -> Bus Creator/9  "Tm (pu)"
  Te/1 -> Bus Creator/10  "Te (pu)"
  Vdq_grid_conv/1 -> Bus Creator/11  "Vdq_grid_conv (pu)"
  Mux2/1 -> Bus Creator/12  "Iabc_grid_conv (cmplx) (pu)"
  Idq_grid_conv/1 -> Bus Creator/13  "Idq_grid_conv (pu)"
  Vdc/1 -> Bus Creator/16  "Vdc (V)"
  -2/1 -> Q_B1/1, Bus Creator/15  "Q (pu)"
  -1/1 -> Bus Creator/14, P_B1/1  "P (pu)"
  Pitch_angle (deg)/1 -> Bus Creator/17  "Pitch_angle (deg)"
  Bus Creator/1 -> m/1
  -->pu1/1 -> -2/1
  "Power (3ph, Phasor)"/1 -> -->pu/1
  "Power (3ph, Phasor)"/2 -> -->pu1/1

== system wind_turbine_modified/Wind Turbine Doubly-Fed Induction Generator (Phasor Type)1/Generator & Converters/Grid-side converter currents & Converters power ==
  Vdq_rotor_conv : Inport
  Vdq_B1 : Inport  Port=2
  Vdq_grid_conv : Inport  Port=3
  Idq_rotor_conv : Inport  Port=4
  Trip : Inport  Port=5
  Demux : Demux  Outputs=2
      settings: DisplayOption=none
  Demux1 : Demux  Outputs=2
      settings: DisplayOption=none
  Mux2 : Mux  Inputs=2
  Product1 : Product  Inputs=**  InputSameDT=on  SaturateOnIntegerOverflow=on  OutDataTypeStr=Inherit: Same as first input
  Product3 : Product  Inputs=**  InputSameDT=on  SaturateOnIntegerOverflow=on  OutDataTypeStr=Inherit: Same as first input
  Sum1 : Sum  Inputs=1  InputSameDT=on  SaturateOnIntegerOverflow=on  OutDataTypeStr=Inherit: Same as first input
  Sum3 : Sum  Inputs=1  InputSameDT=on  SaturateOnIntegerOverflow=on  OutDataTypeStr=Inherit: Same as first input
  d-q axis model of a 3-phase series R-L branch : Subsystem  mask(d-q axis model of a 3-phase series R-L branch){R=R_RL, L=L_RL, Fnom=Fnom, Idq0=[ILd_init ILq_init]}
      mask prompts: R "R (pu)"; L "L (pu)"; Fnom "Nominal frequency (Hz)"; Idq0 "Initial currents [Id Iq] (pu)"
      mask help:
      | This block implements a d-q axis model of a 3-phase R-L branch.
      | Inputs:
      | d-q axis voltages (V1 and V2) at each terminal of the R-L branch in pu.
      | Outputs:
      | d-q axis currents flowing (from V1 to V2) in the R-L branch in pu.
      mask init:
      | w=2*pi*Fnom;
  dq2ab : Subsystem
  Ia_grid_conv : Outport  VectorParamsAs1DForOutWhenUnconnected=off
  Ib_grid_conv : Outport  Port=2  VectorParamsAs1DForOutWhenUnconnected=off
  Idq_grid_conv : Outport  Port=3  VectorParamsAs1DForOutWhenUnconnected=off
  Pac_grid_conv : Outport  Port=4  VectorParamsAs1DForOutWhenUnconnected=off
  Pac_rotor_conv : Outport  Port=5  VectorParamsAs1DForOutWhenUnconnected=off
  wires:
  Demux/2 -> Ib_grid_conv/1
  Demux/1 -> Ia_grid_conv/1
  dq2ab/1(Ia_Ib complx) -> Demux/1
  d-q axis model of a 3-phase series R-L branch/1(Idq) -> dq2ab/1(Idq_seq1), Demux1/1, Product3/1
  Idq_rotor_conv/1 -> Product1/2
  Vdq_rotor_conv/1 -> Product1/1
  Sum1/1 -> Pac_rotor_conv/1
  Product1/1 -> Sum1/1
  Sum3/1 -> Pac_grid_conv/1
  Product3/1 -> Sum3/1
  Vdq_grid_conv/1 -> d-q axis model of a 3-phase series R-L branch/2(Vdq2), Product3/2
  Vdq_B1/1 -> d-q axis model of a 3-phase series R-L branch/1(Vdq1)
  Demux1/1 -> Mux2/1  "Id_grid_conv (pu)"
  Demux1/2 -> Mux2/2  "Iq_grid_conv (pu)"
  Mux2/1 -> Idq_grid_conv/1
  Trip/1 -> d-q axis model of a 3-phase series R-L branch/3(Trip)

== system wind_turbine_modified/Wind Turbine Doubly-Fed Induction Generator (Phasor Type)1/Generator & Converters/Asynchronous machine Positive sequence phasor model Inputs and outputs are in per unit (pu)/Mechanical ==
  Tm : Inport
  phiqds1,iqds1 : Inport  Port=2
  1\p : Gain  Gain=1/p  SaturateOnIntegerOverflow=on  OutDataTypeStr=Inherit: Same as input  ParamDataTypeStr=Inherit: Same as input
  1_2H : Gain  Gain=1/(2*H)  SaturateOnIntegerOverflow=on  OutDataTypeStr=Inherit: Same as input  ParamDataTypeStr=Inherit: Same as input
  F : Gain  Gain=F  SaturateOnIntegerOverflow=on  OutDataTypeStr=Inherit: Same as input  ParamDataTypeStr=Inherit: Same as input
  Integrator : Integrator  InitialCondition=wmo  LowerSaturationLimit=0
  Integrator1 : Integrator  InitialCondition=tho
  Mux4 : Mux  Inputs=3
  Product1 : Product  Inputs=1  InputSameDT=on  SaturateOnIntegerOverflow=on  OutDataTypeStr=Inherit: Same as first input
  Product2 : Product  Inputs=1  InputSameDT=on  SaturateOnIntegerOverflow=on  OutDataTypeStr=Inherit: Same as first input
  Selector : Selector  InputPortWidth=4  IndexOptions=Index vector (dialog)  Indices=[1 4]  OutputSizes=1
  Selector1 : Selector  InputPortWidth=4  IndexOptions=Index vector (dialog)  Indices=[2 3]  OutputSizes=1
  Sum : Sum  Inputs=-+-  InputSameDT=on  SaturateOnIntegerOverflow=on  OutDataTypeStr=Inherit: Same as first input
  Sum1 : Sum  Inputs=|-+  InputSameDT=on  SaturateOnIntegerOverflow=on  OutDataTypeStr=Inherit: Same as first input
  web : Gain  Gain=web  SaturateOnIntegerOverflow=on  OutDataTypeStr=Inherit: Same as input  ParamDataTypeStr=Inherit: Same as input
  wr,Te,thr : Outport  VectorParamsAs1DForOutWhenUnconnected=off
  wires:
  Sum1/1 -> Sum/2, Mux4/2  "Pos.seq.Torque"
  Integrator1/1 -> 1\p/1
  1\p/1 -> Mux4/3
  web/1 -> Integrator1/1
  F/1 -> Sum/3
  Integrator/1 -> web/1, Mux4/1, F/1  "w (pu)"
  1_2H/1 -> Integrator/1
  Sum/1 -> 1_2H/1
  Tm/1 -> Sum/1  "Tm"
  Mux4/1 -> wr,Te,thr/1
  Product1/1 -> Sum1/1
  Product2/1 -> Sum1/2
  phiqds1,iqds1/1 -> Selector/1, Selector1/1
  Selector1/1 -> Product2/1
  Selector/1 -> Product1/1

== system wind_turbine_modified/Wind Turbine Doubly-Fed Induction Generator (Phasor Type)1/Generator & Converters/Asynchronous machine Positive sequence phasor model Inputs and outputs are in per unit (pu)/Phasors Ia Ib stator ==
  note: Ia= I1
  note: Ib= a^2*I1
  note: I1
  Idqs1 : Inport
  Demux : Demux  Outputs=2
      settings: DisplayOption=none
  Mux1 : Mux  Inputs=2
  Mux2 : Mux  Inputs=[2 1]
  Real-Imag to Complex : RealImagToComplex
  Sum : Sum  Inputs=1  InputSameDT=on  SaturateOnIntegerOverflow=on  OutDataTypeStr=Inherit: Same as first input
  a^2 : Gain  Gain=exp(-j*2*pi/3)  SaturateOnIntegerOverflow=on  OutDataTypeStr=Inherit: Same as input  ParamDataTypeStr=Inherit: Same as input
  inv : Gain  Gain=-1  SaturateOnIntegerOverflow=on  OutDataTypeStr=Inherit: Same as input  ParamDataTypeStr=Inherit: Same as input
  Isabc cmplx : Outport  VectorParamsAs1DForOutWhenUnconnected=off
  wires:
  Demux/2 -> Real-Imag to Complex/2
  Demux/1 -> Real-Imag to Complex/1
  a^2/1 -> Mux1/2
  Idqs1/1 -> Demux/1
  Mux1/1 -> Mux2/1, Sum/1  "ia ib"
  Sum/1 -> inv/1
  inv/1 -> Mux2/2  "ic"
  Mux2/1 -> Isabc cmplx/1
  Real-Imag to Complex/1 -> Mux1/1, a^2/1  "I1"

== system wind_turbine_modified/Wind Turbine Doubly-Fed Induction Generator (Phasor Type)1/Generator & Converters/Asynchronous machine Positive sequence phasor model Inputs and outputs are in per unit (pu)/Positive Sequence Model ==
  Vqdr1 : Inport
  w-wr : Inport  Port=2
  Vqds1 : Inport  Port=3
  Trip : Inport  Port=4
  Constant7 : Constant
  Mutual fluxes : Subsystem
  Rotor : Subsystem
      mask Display: disp('Rotor')
  Stator : Subsystem
      mask Display: disp('Stator')
  Iqdr1 : Outport  VectorParamsAs1DForOutWhenUnconnected=off
  Iqds1 : Outport  Port=2  VectorParamsAs1DForOutWhenUnconnected=off
  Phiqds1_Isqds1 : Outport  Port=3  VectorParamsAs1DForOutWhenUnconnected=off
  wires:
  Stator/3(phis,is) -> Phiqds1_Isqds1/1
  Stator/2(iqs,ids) -> Iqds1/1
  w-wr/1 -> Rotor/2(w-wr)
  Rotor/1(iqr,idr) -> Iqdr1/1
  Vqds1/1 -> Stator/2(vqs,vds)
  Vqdr1/1 -> Rotor/1(vqr,vdr)
  Constant7/1 -> Stator/3(w)
  Rotor/2(phiqr,phidr) -> Mutual fluxes/1(phiqr,phidr)
  Stator/1(phiqs,phids) -> Mutual fluxes/2(phiqs,phids)
  Mutual fluxes/1(phimq,phimd) -> Stator/1(phimq,phimd), Rotor/3(phimq,phimd)
  Trip/1 -> Stator/4(Trip), Rotor/4(Trip)

== system wind_turbine_modified/Wind Turbine Doubly-Fed Induction Generator (Phasor Type)1/Generator & Converters/Asynchronous machine Positive sequence phasor model Inputs and outputs are in per unit (pu)/Vab Vbc ==
  Vabc : Inport
  Mux : Mux  Inputs=2
  Selector : Selector  InputPortWidth=3  IndexOptions=Index vector (dialog)  Indices=[1]  OutputSizes=1
  Selector1 : Selector  InputPortWidth=3  IndexOptions=Index vector (dialog)  Indices=[2]  OutputSizes=1
  Selector2 : Selector  InputPortWidth=3  IndexOptions=Index vector (dialog)  Indices=[3]  OutputSizes=1
  Sum : Sum  Inputs=|+-  SaturateOnIntegerOverflow=on
  Sum1 : Sum  Inputs=|+-  SaturateOnIntegerOverflow=on
  Vab_Vbc : Outport  VectorParamsAs1DForOutWhenUnconnected=off
  wires:
  Vabc/1 -> Selector2/1, Selector1/1, Selector/1
  Selector/1 -> Sum/1  "Va"
  Selector1/1 -> Sum/2, Sum1/1  "Vb"
  Sum/1 -> Mux/1  "Vab"
  Selector2/1 -> Sum1/2  "Vc"
  Sum1/1 -> Mux/2  "Vbc"
  Mux/1 -> Vab_Vbc/1

== system wind_turbine_modified/Wind Turbine Doubly-Fed Induction Generator (Phasor Type)1/Generator & Converters/Asynchronous machine Positive sequence phasor model Inputs and outputs are in per unit (pu)/abc2dq ==
  note: V1= 1/3(Vab -a^2*Vbc)
  Vab Vbc cmplx : Inport
  (a^2)/3 : Gain  Gain=1/3*exp(-j*2*pi/3)  SaturateOnIntegerOverflow=on  OutDataTypeStr=Inherit: Same as input  ParamDataTypeStr=Inherit: Same as input
  Complex to Real-Imag : ComplexToRealImag
  Demux : Demux  Outputs=2
      settings: DisplayOption=none
  Gain : Gain  Gain=1/3  SaturateOnIntegerOverflow=on  OutDataTypeStr=Inherit: Same as input  ParamDataTypeStr=Inherit: Same as input
  Mux : Mux  Inputs=2
  Sum3 : Sum  Inputs=+-  InputSameDT=on  SaturateOnIntegerOverflow=on  OutDataTypeStr=Inherit: Same as first input
  Vdqs1 : Outport  VectorParamsAs1DForOutWhenUnconnected=off
  wires:
  Complex to Real-Imag/2 -> Mux/2  "Vq_stator (pu)"
  Complex to Real-Imag/1 -> Mux/1  "Vd_stator (pu)"
  Mux/1 -> Vdqs1/1
  Sum3/1 -> Complex to Real-Imag/1  "V1"
  Demux/1 -> Gain/1
  Vab Vbc cmplx/1 -> Demux/1
  Gain/1 -> Sum3/1
  (a^2)/3/1 -> Sum3/2
  Demux/2 -> (a^2)/3/1

== system wind_turbine_modified/Wind Turbine Doubly-Fed Induction Generator (Phasor Type)1/Generator & Converters/Control/Converters voltages ==
  Vdq_ctrl_grid_conv : Inport
  Vdc : Inport  Port=2
  Vdq_ctrl_rotor_conv : Inport  Port=3
  ->pu : Gain  Gain=1/(Vnom*sqrt(2)/sqrt(3))  SaturateOnIntegerOverflow=on  OutDataTypeStr=Inherit: Same as input  ParamDataTypeStr=Inherit: Same as input
  "->pu " : Gain  Gain=1/(Vnom*sqrt(2)/sqrt(3))  SaturateOnIntegerOverflow=on  OutDataTypeStr=Inherit: Same as input  ParamDataTypeStr=Inherit: Same as input
  Complex to Real-Imag : ComplexToRealImag
  Complex to Real-Imag1 : ComplexToRealImag
  Gain : Gain  Gain=1/2  SaturateOnIntegerOverflow=on  OutDataTypeStr=Inherit: Same as input  ParamDataTypeStr=Inherit: Same as input
  Gain1 : Gain  Gain=1/2  SaturateOnIntegerOverflow=on  OutDataTypeStr=Inherit: Same as input  ParamDataTypeStr=Inherit: Same as input
  Mux1 : Mux  Inputs=2
  Mux2 : Mux  Inputs=2
  Product1 : Product  Inputs=**  InputSameDT=on  SaturateOnIntegerOverflow=on  OutDataTypeStr=Inherit: Same as first input
  Product2 : Product  Inputs=**  InputSameDT=on  SaturateOnIntegerOverflow=on  OutDataTypeStr=Inherit: Same as first input
  Vdq_grid_conv : Outport  VectorParamsAs1DForOutWhenUnconnected=off
  Vdq_rotor_conv : Outport  Port=2  VectorParamsAs1DForOutWhenUnconnected=off
  wires:
  Vdq_ctrl_rotor_conv/1 -> Product1/2
  Vdq_ctrl_grid_conv/1 -> Product2/1
  Product2/1 -> Gain/1
  Product1/1 -> Gain1/1
  Gain/1 -> ->pu/1
  Gain1/1 -> "->pu "/1
  Vdc/1 -> Product1/1, Product2/2
  ->pu/1 -> Complex to Real-Imag/1
  Complex to Real-Imag1/2 -> Mux2/2  "Vq_rotor (pu)"
  Mux2/1 -> Vdq_rotor_conv/1
  Complex to Real-Imag1/1 -> Mux2/1  "Vd_rotor (pu)"
  "->pu "/1 -> Complex to Real-Imag1/1
  Complex to Real-Imag/1 -> Mux1/1  "Vd_grid_conv (pu)"
  Complex to Real-Imag/2 -> Mux1/2  "Vq_grid_conv (pu)"
  Mux1/1 -> Vdq_grid_conv/1

== system wind_turbine_modified/Wind Turbine Doubly-Fed Induction Generator (Phasor Type)1/Generator & Converters/Control/abc2dq & Positive sequence Voltage phase angle ==
  note: V1= 1/3(Va +aVb+a^2*Vc)
  Vabc_B1 : Inport
  (a^2)/3 : Gain  Gain=1/3*exp(-j*2*pi/3)  SaturateOnIntegerOverflow=on  OutDataTypeStr=Inherit: Same as input  ParamDataTypeStr=Inherit: Same as input
  20% : Switch  Threshold=0.5  InputSameDT=off
  Complex to Magnitude-Angle : ComplexToMagnitudeAngle
  Complex to Real-Imag : ComplexToRealImag
  Demux : Demux  Outputs=3
      settings: DisplayOption=none
  Gain : Gain  Gain=1/3  SaturateOnIntegerOverflow=on  OutDataTypeStr=Inherit: Same as input  ParamDataTypeStr=Inherit: Same as input
  IC=ic : Memory  InitialCondition=-pi/2  InheritSampleTime=on
  Magnitude-Angle to Complex : MagnitudeAngleToComplex
  Mux : Mux  Inputs=2
  Relay : Relay  OnSwitchValue=0.5  OffSwitchValue=0.1
  Sum3 : Sum  Inputs=+++  InputSameDT=on  SaturateOnIntegerOverflow=on  OutDataTypeStr=Inherit: Same as first input
  a/3 : Gain  Gain=1/3*exp(j*2*pi/3)  SaturateOnIntegerOverflow=on  OutDataTypeStr=Inherit: Same as input  ParamDataTypeStr=Inherit: Same as input
  Vdq_B1 : Outport  VectorParamsAs1DForOutWhenUnconnected=off
  Theta : Outport  Port=2  VectorParamsAs1DForOutWhenUnconnected=off
  V_B1 : Outport  Port=3  VectorParamsAs1DForOutWhenUnconnected=off
  wires:
  Complex to Real-Imag/2 -> Mux/2  "Vq"
  Complex to Real-Imag/1 -> Mux/1  "Vd"
  Magnitude-Angle to Complex/1 -> Complex to Real-Imag/1
  Complex to Magnitude-Angle/1 -> Relay/1, Magnitude-Angle to Complex/1, V_B1/1
  Sum3/1 -> Complex to Magnitude-Angle/1  "V1"
  (a^2)/3/1 -> Sum3/3
  a/3/1 -> Sum3/2
  Demux/3 -> (a^2)/3/1
  Demux/2 -> a/3/1
  Gain/1 -> Sum3/1
  Vabc_B1/1 -> Demux/1
  Demux/1 -> Gain/1
  Mux/1 -> Vdq_B1/1
  20%/1 -> Theta/1, IC=ic/1
  IC=ic/1 -> 20%/3
  Relay/1 -> 20%/2
  Complex to Magnitude-Angle/2 -> Magnitude-Angle to Complex/2, 20%/1

== system wind_turbine_modified/Wind Turbine Doubly-Fed Induction Generator (Phasor Type)1/Generator & Converters/Control/wind_dfig_grid ==
  note: Grid-side converter control system
  Vdq_B1 : Inport
  Idq_grid_conv : Inport  Port=2
  Theta : Inport  Port=3
  Vdc : Inport  Port=4
  Iq_ref : Inport  Port=5
  Enable : EnablePort  PropagateVarSize=During execution
  Current regulator : Subsystem
  DC bus voltage Regulator : Subsystem
  Idq B1 voltage Reference frame : Subsystem
  Idq references : Subsystem
  Mux : Mux  Inputs=2
  Rate Limiter : RateLimiter  RisingSlewLimit=current_slew_rate  FallingSlewLimit=-current_slew_rate
  Subsystem : Subsystem
  Vdc_ref (V) : Constant  Value=Vdc_nom
  Vdq B1 voltage Reference frame : Subsystem
  Vdq_ctrl_grid_conv : Outport  VectorParamsAs1DForOutWhenUnconnected=off
  wires:
  Iq_ref/1 -> Rate Limiter/1
  Rate Limiter/1 -> Mux/2
  Idq references/1(Idq_ref) -> Current regulator/3(Idq_ref)
  Mux/1 -> Idq references/1(Id*Iq*)
  Idq B1 voltage Reference frame/1(Idq) -> Current regulator/2(Idq)
  DC bus voltage Regulator/1(Id_ref) -> Mux/1
  Idq_grid_conv/1 -> Idq B1 voltage Reference frame/2(Idq_grid_conv)
  Subsystem/1(Vdq_ctrl_grid_conv) -> Vdq_ctrl_grid_conv/1
  Vdc/1 -> DC bus voltage Regulator/2(Vdc), Subsystem/3(Vdc)
  Current regulator/1(Vdq*) -> Subsystem/2(Vdq*)
  Vdc_ref (V)/1 -> DC bus voltage Regulator/1(Vdc_ref)
  Theta/1 -> Subsystem/1(Theta), Vdq B1 voltage Reference frame/1(Theta), Idq B1 voltage Reference frame/1(Theta)
  Vdq_B1/1 -> Vdq B1 voltage Reference frame/2(Vdq_B1)
  Vdq B1 voltage Reference frame/1(Vdq) -> Current regulator/1(Vdq)
